simulink model "photodiode_VEMD2020X01"  (R2024a)
settings: Solver=VariableStepAuto  StartTime=0.0  StopTime=10.0  RelTol=1e-3
undefined symbols (not defined in the file): x, y
libraries: nesl_utility x3, fl_lib x3, simulink x1
settings Model: Creator=tp888  LastModifiedBy=timot

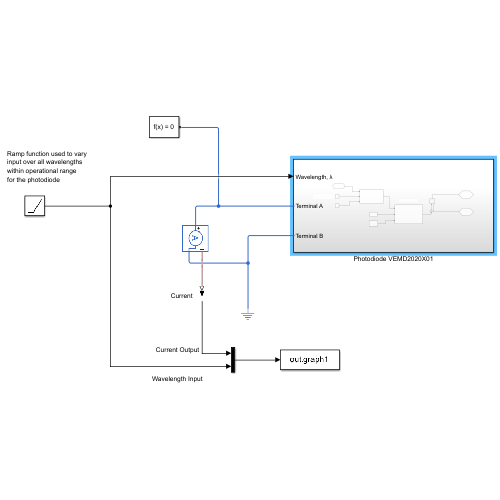
[thumbnail: Simulink's stored preview of the top-level diagram]
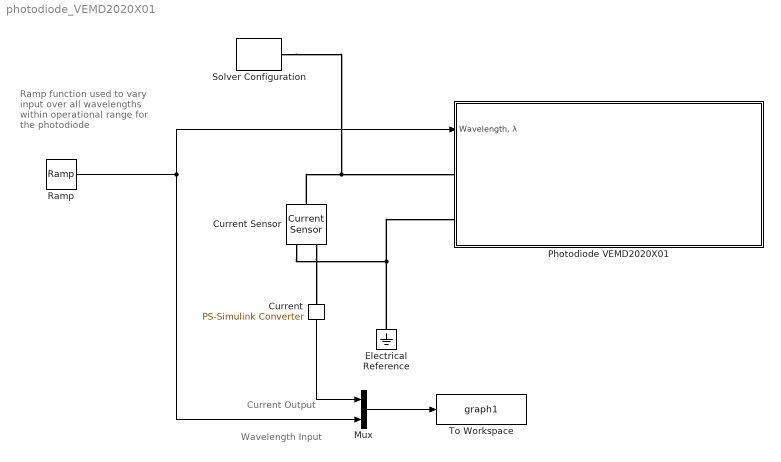
== system photodiode_VEMD2020X01 ==
  note: Ramp function used to vary
      | input over all wavelengths
      | within operational range
      | for the photodiode
  note: Wavelength Input
  note: Current Output
  Current : nesl_utility/PS-Simulink Converter  PhysicalDomain=network_engine_domain  SubClassName=ps_output  LeftPortType=input  RightPortType=output  PseudoPeriodic=off  Frequencies=[]  VectorFormat=inherit  Unit=inherit  AffineConversion=off
  Current Sensor : fl_lib/Electrical/Electrical Sensors/Current Sensor
  Electrical Reference : fl_lib/Electrical/Electrical Elements/Electrical Reference
  Mux : Mux  Inputs=2
  Photodiode VEMD2020X01 : Subsystem
  Ramp : simulink/Sources/Ramp  slope=1.2e-8  start=0  InitialOutput=8.3e-7
  Solver Configuration : nesl_utility/Solver Configuration  PhysicalDomain=network_engine_domain  SubClassName=solver  LeftPortType=input  RightPortType=generic  Tones=[]  Harmonics=[]  SimulateNoise=off  Profile=off  UseLocalSampling=off  EnableSwitchedLinearOptims=on  FrequencyDomain=off  UseCCode=off  RelTol=0.001  AbsTol=0.001  MinStep=1e-09  ToWorkspace=off  RevertToSquareIcSolve=off  NumHomotopyIterations=100  PhasorMode=off  PhasorModeNumHarmonics=1  ConsistencySolver=NEWTON_XTOL_AFTER_FTOL  IndexReductionMethod=DerivativeReplacement  DoDC=off  ResidualTolerance=1e-09  ConsistencyTolSource=GLOBAL  ConsistencyAbsTol=0.001  ConsistencyRelTol=0.001  ConsistencyTolFactor=0.001  UseLocalSolver=off  LocalSolverChoice=NE_BACKWARD_EULER_ADVANCER  ResolveIndetEquations=on  FunctionEvalNumThread=1  LocalSolverSampleTime=0.001  DoFixedCost=off  MaxNonlinIter=3  MaxModeIter=2  ComputeImpulses=off  ImpulseIterations=2  LinearAlgebra=auto  LinearAlgebraNumThread=0  EquationFormulation=NE_TIME_EF  DelaysMemoryBudget=1024  AutomaticFiltering=on  FilteringTimeConstant=0.001  PartitionStorageMethod=AS_NEEDED  PartitionMemoryBudget=1024  PartitionMethod=ROBUST  MultibodyUseLocalSolver=off  MultibodyLocalSolverChoice=ODE1  MultibodyLocalSolverSampleTime=0.001
  To Workspace : ToWorkspace  VariableName=graph1  SaveFormat=Timeseries  SampleTime=-1
  wires:
  Ramp/1 -> Photodiode VEMD2020X01/1("Wavelength, λ"), Mux/2
  Mux/1 -> To Workspace/1
  Current/1 -> Mux/1
  connections:
  Electrical Reference/LConn1 -- Current Sensor/RConn2 -- Photodiode VEMD2020X01/LConn2
  Solver Configuration/RConn1 -- Current Sensor/LConn1 -- Photodiode VEMD2020X01/LConn1
  Current Sensor/RConn1 -- Current/LConn1

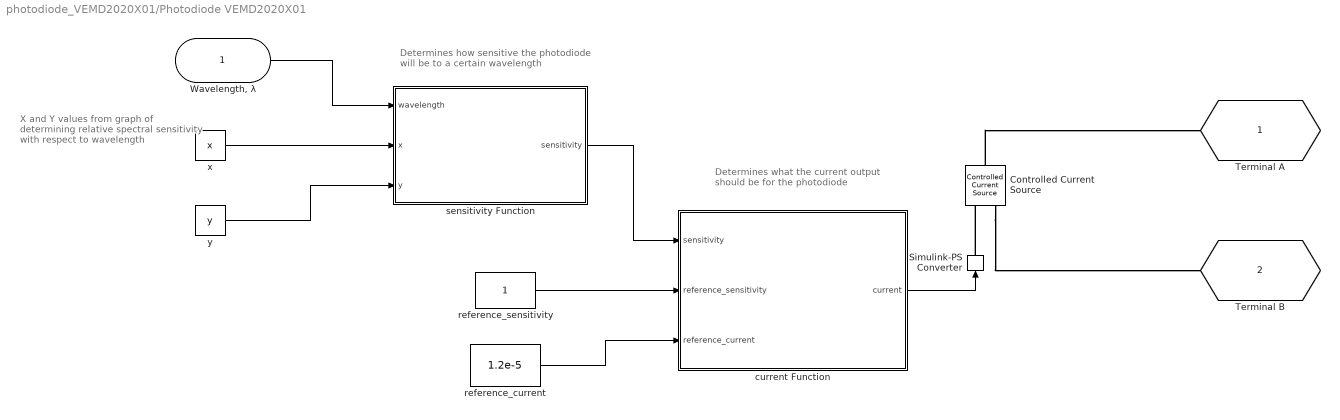
== system photodiode_VEMD2020X01/Photodiode VEMD2020X01 ==
  note: Determines what the current
      | output should be for the photodiode
  note: Determines how sensitive the photodiode
      | will be to a certain wavelength
  note: X and Y values from graph of
      | determining relative spectral
      | sensitivity with respect to wavelength
  "Wavelength, λ" : Inport
  Controlled Current Source : fl_lib/Electrical/Electrical Sources/Controlled Current Source
  Simulink-PS Converter : nesl_utility/Simulink-PS Converter  PhysicalDomain=network_engine_domain  SubClassName=ps_input  LeftPortType=input  RightPortType=output  PseudoPeriodic=off  Frequencies=[]  NoiseDistribution=none  NoiseParameters=[]  Unit=1  AffineConversion=off  FilteringAndDerivatives=provide  SimscapeFilterOrder=1  InputFilterTimeConstant=0.001  UdotUserProvided=0
  current Function : MATLAB Function  TreatAsAtomicUnit=on
  reference_current : Constant  Value=1.2e-5
  reference_sensitivity : Constant
  sensitivity Function : MATLAB Function  TreatAsAtomicUnit=on
  x : Constant  Value=x
  y : Constant  Value=y
  Terminal A : PMIOPort  Side=Left
  Terminal B : PMIOPort  Port=2  Side=Left
  wires:
  sensitivity Function/1(sensitivity) -> current Function/1(sensitivity)
  x/1 -> sensitivity Function/2(x)
  current Function/1(current) -> Simulink-PS Converter/1
  reference_sensitivity/1 -> current Function/2(reference_sensitivity)
  reference_current/1 -> current Function/3(reference_current)
  y/1 -> sensitivity Function/3(y)
  "Wavelength, λ"/1 -> sensitivity Function/1(wavelength)
  connections:
  Simulink-PS Converter/RConn1 -- Controlled Current Source/RConn1
  Controlled Current Source/RConn2 -- Terminal B/RConn1
  Controlled Current Source/LConn1 -- Terminal A/RConn1

== matlab function photodiode_VEMD2020X01/Photodiode VEMD2020X01/current Function ==
  data: sensitivity input; current output; reference_sensitivity input; reference_current input
function current = current(sensitivity, reference_sensitivity, reference_current)

%Determines current based on sensitivity of the photodiode to a wavelength

current = reference_current * (sensitivity/reference_sensitivity);

== matlab function photodiode_VEMD2020X01/Photodiode VEMD2020X01/sensitivity Function ==
  data: wavelength input; sensitivity output; x input; y input
function sensitivity = sensitivity(wavelength, x, y)

%Ensures wavelength is within operational range for photodiode
if wavelength < 8.3e-7
    error("Invalid wavelength");
elseif wavelength > 9.5e-7
    error("Invalid wavelength");
end

%Interpolates the sensitivtiy based on graph from datasheet
persistent interpFunc;
if isempty(interpFunc)
    interpFunc = @(xq) interp1(x, y, xq, 'linear');
end

sensitivity = interpFunc(wavelength);
end
